simulink model "PID_Real_Time_System"  (R2018b)
settings: Solver=FixedStepAuto  StartTime=0.0  StopTime=inf  RelTol=1e-3  EnableMultiTasking=on
undefined symbols (not defined in the file): h, kd, ki, kp, serial
libraries: instrumentlib x3
settings Model: ExtModeTrigDuration=2  Creator=fred  LastModifiedBy=fredericovaz
settings SolverCC: AutoInsertRateTranBlk=on
settings OptimizationCC: EnhancedBackFolding=on  PassReuseOutputArgsAs=Individual arguments  MaxStackSize=64  OptimizeBlockOrder=speed  DifferentSizesBufferReuse=on  OptimizationCustomize=off
settings DebuggingCC: ParameterTunabilityLossMsg=error
settings HardwareCC: ProdBitPerInt=16  ProdBitPerPointer=16  ProdBitPerSizeT=16  ProdBitPerPtrDiffT=16  ProdLargestAtomicFloat=None  ProdWordSize=8  ProdHWDeviceType=Atmel->AVR  UseEmbeddedCoderFeatures=off
settings SFSimCC: MATLABDynamicMemAlloc=off
settings RTWCC: SystemTargetFile=ert.tlc  HardwareBoard=Arduino Mega 2560  TemplateMakefile=ert_default_tmf  GenerateReport=on  Toolchain=Arduino AVR  BuildConfiguration=Faster Runs  IncludeHyperlinkInReport=on  LaunchReport=on  GenerateTraceInfo=on  GenerateTraceReport=on  GenerateTraceReportSl=on  GenerateTraceReportSf=on  GenerateTraceReportEml=on
settings CodeAppCC: ForceParamTrailComments=on  IgnoreCustomStorageClasses=off  OperatorAnnotations=on  SimulinkDataObjDesc=on  SFDataObjDesc=on  InsertBlockDesc=on
settings ERTTargetCC: SupportContinuousTime=on  SupportNonInlinedSFcns=on  SupportVariableSizeSignals=on

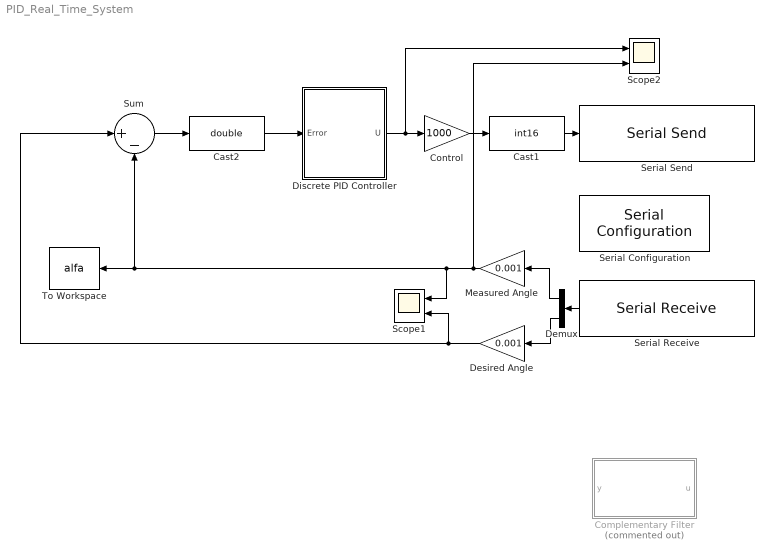
== system PID_Real_Time_System ==
  Cast1 : DataTypeConversion  OutDataTypeStr=int16
  Cast2 : DataTypeConversion  OutDataTypeStr=double
  Complementary Filter : MATLAB Function  Commented=on  TreatAsAtomicUnit=on
  Control : Gain  Gain=1000
  Demux : Demux  Outputs=2
  Desired Angle : Gain  Gain=0.001
  Discrete PID Controller : Subsystem
  Measured Angle : Gain  Gain=0.001
  Scope1 : Scope  NumInputPorts=2
  Scope2 : Scope  NumInputPorts=2
  Serial Configuration : instrumentlib/Serial Configuration  Priority=-200000  ComPortMenu=/dev/cu.usbmodem14101  ComPort=/dev/cu.usbmodem14101  ObjConstructor=serial('/dev/cu.usbmodem14101');  BaudRate=115200  DataBits=8  Parity=none  StopBits=1  FlowControl=none  Timeout=10  ByteOrder=LittleEndian
  Serial Receive : instrumentlib/Serial Receive  ComPortMenu=/dev/cu.usbmodem14101  ComPort=/dev/cu.usbmodem14101  ObjConstructor=serial('/dev/cu.usbmodem14101');  Terminator=<none>  DataSize=2  DataType=int16  EnableBlockingMode=on  ActionDataUnavailable=Output last received value  CustomValue=0  SampleTime=h
  Serial Send : instrumentlib/Serial Send  ComPortMenu=/dev/cu.usbmodem14101  ComPort=/dev/cu.usbmodem14101  ObjConstructor=serial('/dev/cu.usbmodem14101');  Terminator=<none>  EnableBlockingMode=on
  Sum : Sum  Inputs=|+-
  To Workspace : ToWorkspace  VariableName=alfa  SaveFormat=Timeseries  SampleTime=-1
      settings: Save2DSignal=2-D array (concatenate along first dimension)
  wires:
  Discrete PID Controller/1(U) -> Scope2/1, Control/1
  Cast1/1 -> Serial Send/1
  Demux/2 -> Desired Angle/1
  Demux/1 -> Measured Angle/1
  Serial Receive/1 -> Demux/1
  Measured Angle/1 -> Scope1/1, Sum/2, To Workspace/1, Scope2/2
  Desired Angle/1 -> Scope1/2, Sum/1
  Cast2/1 -> Discrete PID Controller/1(Error)
  Sum/1 -> Cast2/1
  Control/1 -> Cast1/1

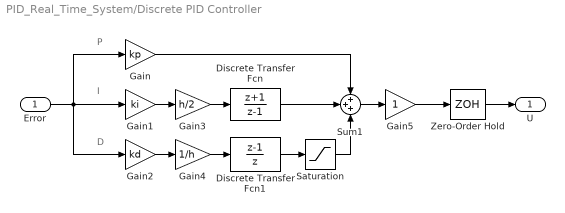
== system PID_Real_Time_System/Discrete PID Controller ==
  note: I
  note: D
  note: P
  Error : Inport
  Discrete Transfer Fcn : DiscreteTransferFcn  Numerator=[1 +1]  Denominator=[1 -1]  SampleTime=h
  Discrete Transfer Fcn1 : DiscreteTransferFcn  Numerator=[1 -1]  Denominator=[1 0]  SampleTime=h
  Gain : Gain  Gain=kp
  Gain1 : Gain  Gain=ki
  Gain2 : Gain  Gain=kd
  Gain3 : Gain  Gain=h/2
  Gain4 : Gain  Gain=1/h
  Gain5 : Gain
  Saturation : Saturate  UpperLimit=8  LowerLimit=-8
  Sum1 : Sum  Inputs=+++
  Zero-Order Hold : ZeroOrderHold  SampleTime=h
  U : Outport
  wires:
  Gain1/1 -> Gain3/1
  Error/1 -> Gain1/1, Gain2/1, Gain/1
  Zero-Order Hold/1 -> U/1
  Sum1/1 -> Gain5/1
  Gain2/1 -> Gain4/1
  Gain/1 -> Sum1/1
  Gain3/1 -> Discrete Transfer Fcn/1
  Discrete Transfer Fcn/1 -> Sum1/2
  Gain4/1 -> Discrete Transfer Fcn1/1
  Discrete Transfer Fcn1/1 -> Saturation/1
  Gain5/1 -> Zero-Order Hold/1
  Saturation/1 -> Sum1/3

== matlab function PID_Real_Time_System/Complementary Filter ==
  data: u input; y output
function y = fcn(u)

y = u;
